simulink model "Bud3_wezel1_2010"  (R2024b)
settings: Solver=ode45  StartTime=0.0  StopTime=1000  MaxStep=0.1  RelTol=1e-3  EnableMultiTasking=on
values from neighbouring files (symbols this model uses):
  atz_c = (TwzN-TzewN)/(TwewN-TzewN)    (= 3.75)    [project1.m]
  btz_c = (TwzN-TwewN)/(TwewN-TzewN)    (= 2.75)    [project1.m]
  cpw = 4200    [project1.m]
  Cw = cpw*row*Vw  / skala    (= 700)    [project1.m]
  czas_skok = 100    [project1.m]
  dFg = [0, 0, 0] .* FgN    [project1.m]
  dFw = 0.1 * FwN    [project1.m]
  dQd = [0, 0, 0] .* QN    [project1.m]
  dSPc = 0    [project1.m]
  dTwz = 0    [project1.m]
  dTzew = 0    [project1.m]
  Fg0 = [1, 1, 1] .* FgN    [project1.m]
  Fw0 = tabFw0(ipp)    [project1.m]
  k = 1 / (0.1*FwN)    [project1.m]
  Kco = QwN / (TwpN - TozN)    [project1.m]
  KPc = 1    [project1.m]
  Qd0 = [0, 0, 0]    [project1.m]
  SPc0 = TwewN    (= 20)    [project1.m]
  T = 1000    [project1.m]
  T0 = 100    [project1.m]
  tau_cieplownia = 60*60 / skala    (= 60)    [project1.m]
  Tgp032 = (Tgp0(3)*Fg0(3) + Tgp0(2)*Fg0(2)  )   /   (  Fg0(3)+Fg0(2)    )    [project1.m]
  Tgp0321 = (Tgp0(3)*Fg0(3) + Tgp0(2)*Fg0(2)  + Tgp0(1)*Fg0(1)  )   /   (  Fg0(3) + Fg0(2) + Fg0(1)    )    [project1.m]
  Toz0 = x0( IlePom*2+1)    [project1.m]
  Twp0 = x0( IlePom*2+2)    [project1.m]
  Twz0 = tabTwz0(ipp)    [project1.m]
  Tzew0 = tabTzew0(ipp)    [project1.m]
undefined symbols (not defined in the file or in its folder): Cg, Cp, Kg, Kstr, T0_s, Tgp0, Twew0
settings Model: Creator=Mateusz  LastModifiedBy=Adam
settings SolverCC: AlgebraicLoopSolver=TrustRegion
settings DataIOCC: LimitDataPoints=on  SaveFormat=Array  SignalLoggingSaveFormat=ModelDataLogs  ReturnWorkspaceOutputs=off
settings OptimizationCC: ExpressionDepthLimit=2147483647  LifeSpan=inf
settings DebuggingCC: UnderspecifiedInitializationDetection=Classic  MergeDetectMultiDrivingBlocksExec=none  SolverPrmCheckMsg=warning  FcnCallInpInsideContextMsg=warning  UnconnectedInputMsg=warning  UnconnectedOutputMsg=warning  UnconnectedLineMsg=warning  StateNameClashWarn=warning  SFUnexpectedBacktrackingDiag=warning  SFNoUnconditionalDefaultTransitionDiag=warning  SFExecutionAtInitializationDiag=none  ArithmeticOperatorsInVariantConditions=warning
settings HardwareCC: ProdBitPerPointer=32  ProdBitPerSizeT=32  ProdBitPerPtrDiffT=32  ProdLargestAtomicFloat=None  ProdIntDivRoundTo=Undefined  ProdEndianess=Unspecified  ProdWordSize=32  ProdHWDeviceType=32-bit Generic
settings ModelReferenceCC: PropagateSignalLabelsOutOfModel=off
settings SFSimCC: SimUseLocalCustomCode=off  CustomCodeUndefinedFunction=UseInterfaceOnly
settings RTWCC: RTWUseLocalCustomCode=off  GPUComputeCapability=3.5
settings CodeAppCC: StateflowObjectComments=on
settings GRTTargetCC: TargetLangStandard=C89/C90 (ANSI)  CombineOutputUpdateFcns=off  GRTInterface=on
settings ConfigComp: CovMetricSettings=dw  CovSaveCumulativeToWorkspaceVar=on  CovSaveSingleToWorkspaceVar=on  CovExternalEMLEnable=off

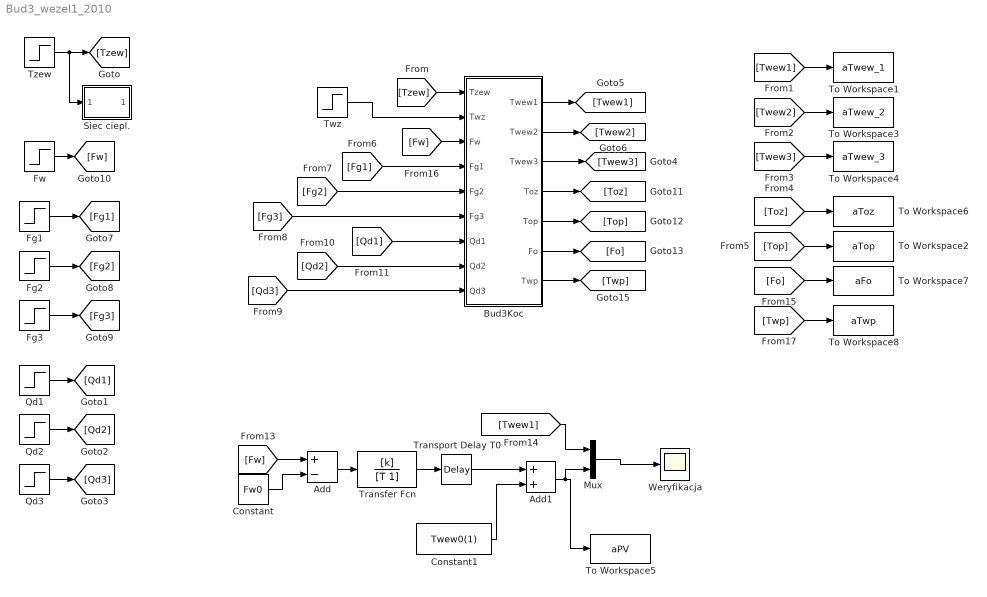
== system Bud3_wezel1_2010 ==
  Add : Sum  Inputs=+-
  Add1 : Sum
  Bud3Koc : Subsystem
  Constant : Constant  Value=Fw0
  Constant1 : Constant  Value=Twew0(1)
  Fg1 : Step  Time=czas_skok  Before=Fg0(1)  After=Fg0(1)+dFg(1)  SampleTime=0
  Fg2 : Step  Time=czas_skok  Before=Fg0(2)  After=Fg0(2)+dFg(2)  SampleTime=0
  Fg3 : Step  Time=czas_skok  Before=Fg0(3)  After=Fg0(3)+dFg(3)  SampleTime=0
  Fw : Step  Time=czas_skok  Before=Fw0  After=Fw0+dFw  SampleTime=0
  Mux : Mux  Inputs=2
  Qd1 : Step  Time=czas_skok  Before=Qd0(1)  After=Qd0(1)+dQd(1)  SampleTime=0
  Qd2 : Step  Time=czas_skok  Before=Qd0(2)  After=Qd0(2)+dQd(2)  SampleTime=0
  Qd3 : Step  Time=czas_skok  Before=Qd0(3)  After=Qd0(3)+dQd(3)  SampleTime=0
  Siec ciepl. : Subsystem
  To Workspace1 : ToWorkspace  VariableName=aTwew_1  SampleTime=-1
  To Workspace2 : ToWorkspace  VariableName=aTop  SampleTime=-1
  To Workspace3 : ToWorkspace  VariableName=aTwew_2  SampleTime=-1
  To Workspace4 : ToWorkspace  VariableName=aTwew_3  SampleTime=-1
  To Workspace5 : ToWorkspace  VariableName=aPV  SampleTime=-1
  To Workspace6 : ToWorkspace  VariableName=aToz  SampleTime=-1
  To Workspace7 : ToWorkspace  VariableName=aFo  SampleTime=-1
  To Workspace8 : ToWorkspace  VariableName=aTwp  SampleTime=-1
  Transfer Fcn : TransferFcn  Numerator=[k]  Denominator=[T 1]
  Transport Delay T0 : TransportDelay  DelayTime=T0
  Twz : Step  Time=czas_skok  Before=Twz0  After=Twz0 + dTwz  SampleTime=0
  Tzew : Step  Time=czas_skok  Before=Tzew0  After=Tzew0+dTzew  SampleTime=0
  Weryfikacja : Scope
  wires:
  Tzew/1 -> [Tzew], Siec ciepl./1(Tzew)
  Fg1/1 -> [Fg1]
  Fg2/1 -> [Fg2]
  Fg3/1 -> [Fg3]
  Fw/1 -> [Fw]
  Transfer Fcn/1 -> Transport Delay T0/1
  Add/1 -> Transfer Fcn/1
  [Fw] -> Add/1
  Constant/1 -> Add/2
  [Twew1] -> Mux/1
  Mux/1 -> Weryfikacja/1
  Transport Delay T0/1 -> Add1/1
  Add1/1 -> Mux/2, To Workspace5/1
  Constant1/1 -> Add1/2
  Bud3Koc/1(Twew1) -> [Twew1]
  Bud3Koc/2(Twew2) -> [Twew2]
  Twz/1 -> Bud3Koc/2(Twz)
  [Tzew] -> Bud3Koc/1(Tzew)
  [Fg1] -> Bud3Koc/4(Fg1)
  [Fg2] -> Bud3Koc/5(Fg2)
  [Fg3] -> Bud3Koc/6(Fg3)
  Qd1/1 -> [Qd1]
  Qd2/1 -> [Qd2]
  Qd3/1 -> [Qd3]
  [Twew1] -> To Workspace1/1
  [Twew2] -> To Workspace3/1
  [Twew3] -> To Workspace4/1
  Bud3Koc/4(Toz) -> [Toz]
  Bud3Koc/5(Top) -> [Top]
  [Toz] -> To Workspace6/1
  [Top] -> To Workspace2/1
  [Qd3] -> Bud3Koc/9(Qd3)
  [Qd2] -> Bud3Koc/8(Qd2)
  [Qd1] -> Bud3Koc/7(Qd1)
  Bud3Koc/6(Fo) -> [Fo]
  [Fo] -> To Workspace7/1
  Bud3Koc/3(Twew3) -> [Twew3]
  [Fw] -> Bud3Koc/3(Fw)
  [Twp] -> To Workspace8/1
  Bud3Koc/7(Twp) -> [Twp]

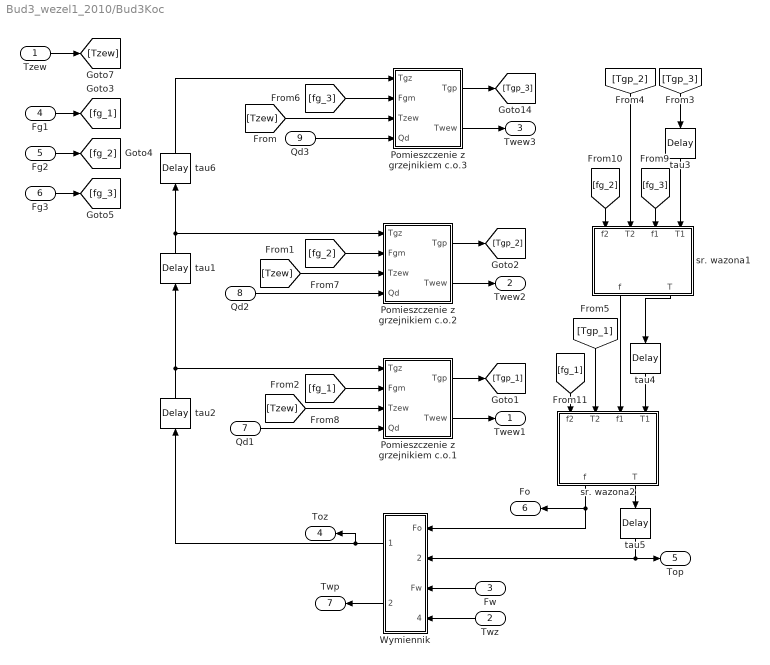
== system Bud3_wezel1_2010/Bud3Koc ==
  Tzew : Inport
  Twz : Inport  Port=2
  Fw : Inport  Port=3
  Fg1 : Inport  Port=4
  Fg2 : Inport  Port=5
  Fg3 : Inport  Port=6
  Qd1 : Inport  Port=7
  Qd2 : Inport  Port=8
  Qd3 : Inport  Port=9
  Pomieszczenie z grzejnikiem c.o.1 : Subsystem  mask{kg=Kg(1), kstr=Kstr(1), Cg=Cg(1), Cp=Cp(1), Tgp0=Tgp0(1), Twew0=Twew0(1), cpw=cpw}
      mask prompts: kg "Wspolczynnik strat ciepla scian grzejnika"; kstr "Wspolczynnik strat ciepla scian pomieszczenia"; Cg "Pojemnosc cieplna grzejnika"; Cp "Pojemnosc cieplna pomieszczenia"; Tgp0 "Temperatura poczatkowa wody powracajacej"; Twew0 "Temperatura poczatkowa wewnatrz pomieszczenia"; cpw "Cieplo wlasciwe"
      mask init:
      | cpw=4200;
      | row=1000;
  Pomieszczenie z grzejnikiem c.o.2 : Subsystem  mask{kg=Kg(2), kstr=Kstr(2), Cg=Cg(2), Cp=Cp(2), Tgp0=Tgp0(2), Twew0=Twew0(2), cpw=cpw}
      mask prompts: kg "Wspolczynnik strat ciepla scian grzejnika"; kstr "Wspolczynnik strat ciepla scian pomieszczenia"; Cg "Pojemnosc cieplna grzejnika"; Cp "Pojemnosc cieplna pomieszczenia"; Tgp0 "Temperatura poczatkowa wody powracajacej"; Twew0 "Temperatura poczatkowa wewnatrz pomieszczenia"; cpw "Cieplo wlasciwe"
      mask init:
      | cpw=4200;
      | row=1000;
  Pomieszczenie z grzejnikiem c.o.3 : Subsystem  mask{kg=Kg(3), kstr=Kstr(3), Cg=Cg(3), Cp=Cp(3), Tgp0=Tgp0(3), Twew0=Twew0(3), cpw=cpw}
      mask prompts: kg "Wspolczynnik strat ciepla scian grzejnika"; kstr "Wspolczynnik strat ciepla scian pomieszczenia"; Cg "Pojemnosc cieplna grzejnika"; Cp "Pojemnosc cieplna pomieszczenia"; Tgp0 "Temperatura poczatkowa wody powracajacej"; Twew0 "Temperatura poczatkowa wewnatrz pomieszczenia"; cpw "Cieplo wlasciwe"
      mask init:
      | cpw=4200;
      | row=1000;
  Wymiennik : Subsystem  mask{cpw=cpw, Kcc=Kco, Cv1=Cw, Cv2=Cw, Twp0=Twp0, Toz0=Toz0}
      mask prompts: Cv1 "Cv1 (str.zasilania)"; Cv2 "Cv2 (str.odbiornik)"
  sr. wazona1 : Subsystem
  sr. wazona2 : Subsystem
  tau1 : TransportDelay  DelayTime=T0_s(2)  InitialOutput=Toz0
  tau2 : TransportDelay  DelayTime=T0_s(1)  InitialOutput=Toz0
  tau3 : TransportDelay  DelayTime=T0_s(3)  InitialOutput=Tgp0(3)
  tau4 : TransportDelay  DelayTime=T0_s(2)  InitialOutput=Tgp032
  tau5 : TransportDelay  DelayTime=T0_s(1)  InitialOutput=Tgp0321
  tau6 : TransportDelay  DelayTime=T0_s(3)  InitialOutput=Toz0
  Twew1 : Outport
  Twew2 : Outport  Port=2
  Twew3 : Outport  Port=3
  Toz : Outport  Port=4
  Top : Outport  Port=5
  Fo : Outport  Port=6
  Twp : Outport  Port=7
  wires:
  tau1/1 -> Pomieszczenie z grzejnikiem c.o.2/1(Tgz), tau6/1
  tau2/1 -> Pomieszczenie z grzejnikiem c.o.1/1(Tgz), tau1/1
  Wymiennik/1(Toz) -> tau2/1, Toz/1
  Qd2/1 -> Pomieszczenie z grzejnikiem c.o.2/4(Qd)
  sr. wazona1/2(T) -> tau4/1
  tau3/1 -> sr. wazona1/4(T1)
  sr. wazona2/2(T) -> tau5/1
  tau5/1 -> Top/1, Wymiennik/2(Top)
  sr. wazona2/1(f) -> Fo/1, Wymiennik/1(Fo)
  tau4/1 -> sr. wazona2/4(T1)
  sr. wazona1/1(f) -> sr. wazona2/3(f1)
  [Tzew] -> Pomieszczenie z grzejnikiem c.o.2/3(Tzew)
  Pomieszczenie z grzejnikiem c.o.1/1(Tgp) -> [Tgp_1]
  Pomieszczenie z grzejnikiem c.o.2/1(Tgp) -> [Tgp_2]
  [Tgp_3] -> tau3/1
  [Tgp_2] -> sr. wazona1/2(T2)
  [Tgp_1] -> sr. wazona2/2(T2)
  [fg_3] -> sr. wazona1/3(f1)
  [fg_2] -> sr. wazona1/1(f2)
  [fg_1] -> sr. wazona2/1(f2)
  Tzew/1 -> [Tzew]
  Pomieszczenie z grzejnikiem c.o.1/2(Twew) -> Twew1/1
  Pomieszczenie z grzejnikiem c.o.2/2(Twew) -> Twew2/1
  Qd1/1 -> Pomieszczenie z grzejnikiem c.o.1/4(Qd)
  [Tzew] -> Pomieszczenie z grzejnikiem c.o.1/3(Tzew)
  Pomieszczenie z grzejnikiem c.o.3/1(Tgp) -> [Tgp_3]
  Pomieszczenie z grzejnikiem c.o.3/2(Twew) -> Twew3/1
  Qd3/1 -> Pomieszczenie z grzejnikiem c.o.3/4(Qd)
  [Tzew] -> Pomieszczenie z grzejnikiem c.o.3/3(Tzew)
  tau6/1 -> Pomieszczenie z grzejnikiem c.o.3/1(Tgz)
  Fg1/1 -> [fg_1]
  Fg2/1 -> [fg_2]
  Fg3/1 -> [fg_3]
  [fg_3] -> Pomieszczenie z grzejnikiem c.o.3/2(Fgm)
  [fg_2] -> Pomieszczenie z grzejnikiem c.o.2/2(Fgm)
  [fg_1] -> Pomieszczenie z grzejnikiem c.o.1/2(Fgm)
  Wymiennik/2(Twp) -> Twp/1
  Fw/1 -> Wymiennik/3(Fw)
  Twz/1 -> Wymiennik/4(Twz)

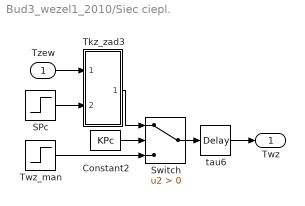
== system Bud3_wezel1_2010/Siec ciepl. ==
  Tzew : Inport
  Constant2 : Constant  Value=KPc
  SPc : Step  Time=czas_skok  Before=SPc0  After=SPc0+dSPc  SampleTime=0
  Switch : Switch  Criteria=u2 > Threshold  SaturateOnIntegerOverflow=off  InputSameDT=off
  Tkz_zad3 : Subsystem  mask{atp=atz_c, btp=btz_c}
      mask prompts: atp "atp (*Tw)"; btp "btp (*Tz)"
  Twz_man : Step  Time=czas_skok  Before=Twz0  After=Twz0+dTwz  SampleTime=0
  tau6 : TransportDelay  DelayTime=tau_cieplownia  InitialOutput=Twz0
  Twz : Outport
  wires:
  SPc/1 -> Tkz_zad3/2(Tw_zad)
  Tkz_zad3/1(Tsz) -> Switch/1
  Twz_man/1 -> Switch/3
  Constant2/1 -> Switch/2
  Switch/1 -> tau6/1
  Tzew/1 -> Tkz_zad3/1(Tzew)
  tau6/1 -> Twz/1

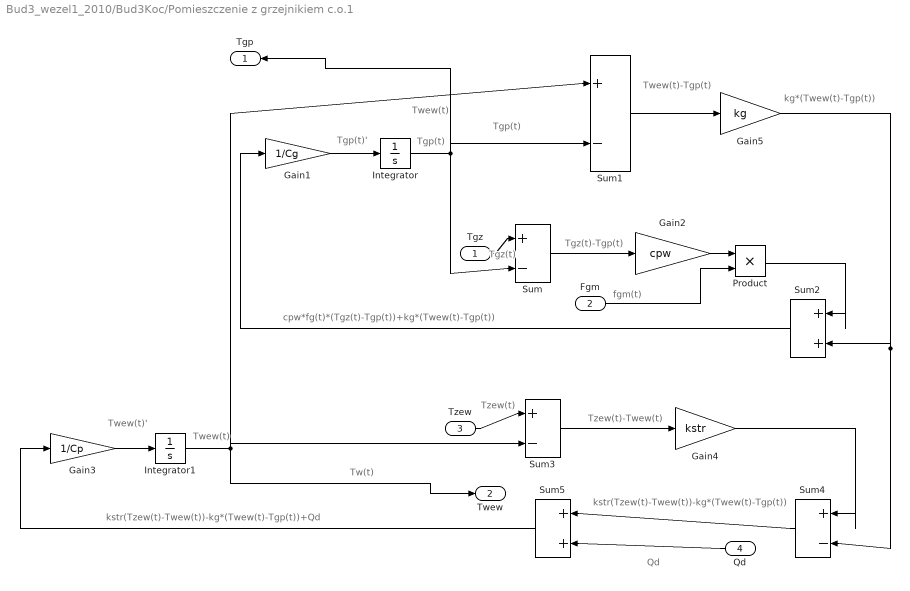
== system Bud3_wezel1_2010/Bud3Koc/Pomieszczenie z grzejnikiem c.o.1 ==
  note: Tgp(t)'
  note: Tgp(t)
  note: Tgz(t)-Tgp(t)
  note: fgm(t)
  note: Tgz(t)
  note: Twew(t)'
  note: Twew(t)
  note: Tzew(t)-Twew(t)
  note: Tzew(t)
  note: Twew(t)-Tgp(t)
  note: Twew(t)
  note: Tw(t)
  note: Tgp(t)
  note: Qd
  note: kg*(Twew(t)-Tgp(t))
  note: cpw*fg(t)*(Tgz(t)-Tgp(t))+kg*(Twew(t)-Tgp(t))
  note: kstr(Tzew(t)-Twew(t))-kg*(Twew(t)-Tgp(t))
  note: kstr(Tzew(t)-Twew(t))-kg*(Twew(t)-Tgp(t))+Qd
  Tgz : Inport
  Fgm : Inport  Port=2
  Tzew : Inport  Port=3
  Qd : Inport  Port=4
  Gain1 : Gain  Gain=1/Cg
  Gain2 : Gain  Gain=cpw
  Gain3 : Gain  Gain=1/Cp
  Gain4 : Gain  Gain=kstr
  Gain5 : Gain  Gain=kg
  Integrator : Integrator  InitialCondition=Tgp0
  Integrator1 : Integrator  InitialCondition=Twew0
  Product : Product  RndMeth=Zero
  Sum{,1,3..4} (4 alike) : Sum  Inputs=|+-
  Sum2 : Sum  Inputs=|++
  Sum5 : Sum  Inputs=|++
  Tgp : Outport
  Twew : Outport  Port=2
  wires:
  Integrator/1 -> Sum/2, Sum1/2, Tgp/1
  Tgz/1 -> Sum/1
  Gain1/1 -> Integrator/1
  Sum/1 -> Gain2/1
  Sum1/1 -> Gain5/1
  Fgm/1 -> Product/2
  Integrator1/1 -> Sum1/1, Sum3/2, Twew/1
  Gain3/1 -> Integrator1/1
  Sum3/1 -> Gain4/1
  Gain5/1 -> Sum2/2, Sum4/2
  Tzew/1 -> Sum3/1
  Sum5/1 -> Gain3/1
  Sum2/1 -> Gain1/1
  Product/1 -> Sum2/1
  Gain4/1 -> Sum4/1
  Qd/1 -> Sum5/2
  Sum4/1 -> Sum5/1
  Gain2/1 -> Product/1

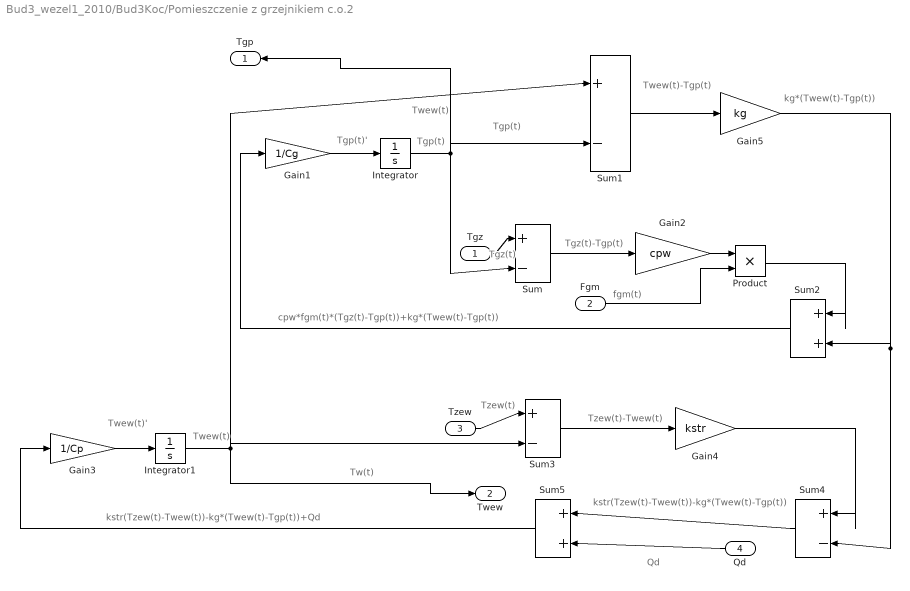
== system Bud3_wezel1_2010/Bud3Koc/Pomieszczenie z grzejnikiem c.o.2 ==
  note: Tgp(t)'
  note: Tgp(t)
  note: Tgz(t)-Tgp(t)
  note: fgm(t)
  note: Tgz(t)
  note: Twew(t)'
  note: Twew(t)
  note: Tzew(t)-Twew(t)
  note: Tzew(t)
  note: Twew(t)-Tgp(t)
  note: Twew(t)
  note: Tw(t)
  note: Tgp(t)
  note: Qd
  note: kg*(Twew(t)-Tgp(t))
  note: cpw*fgm(t)*(Tgz(t)-Tgp(t))+kg*(Twew(t)-Tgp(t))
  note: kstr(Tzew(t)-Twew(t))-kg*(Twew(t)-Tgp(t))
  note: kstr(Tzew(t)-Twew(t))-kg*(Twew(t)-Tgp(t))+Qd
  Tgz : Inport
  Fgm : Inport  Port=2
  Tzew : Inport  Port=3
  Qd : Inport  Port=4
  Gain1 : Gain  Gain=1/Cg
  Gain2 : Gain  Gain=cpw
  Gain3 : Gain  Gain=1/Cp
  Gain4 : Gain  Gain=kstr
  Gain5 : Gain  Gain=kg
  Integrator : Integrator  InitialCondition=Tgp0
  Integrator1 : Integrator  InitialCondition=Twew0
  Product : Product  RndMeth=Zero
  Sum{,1,3..4} (4 alike) : Sum  Inputs=|+-
  Sum2 : Sum  Inputs=|++
  Sum5 : Sum  Inputs=|++
  Tgp : Outport
  Twew : Outport  Port=2
  wires:
  Integrator/1 -> Sum/2, Sum1/2, Tgp/1
  Tgz/1 -> Sum/1
  Gain1/1 -> Integrator/1
  Sum/1 -> Gain2/1
  Sum1/1 -> Gain5/1
  Fgm/1 -> Product/2
  Integrator1/1 -> Sum1/1, Sum3/2, Twew/1
  Gain3/1 -> Integrator1/1
  Sum3/1 -> Gain4/1
  Gain5/1 -> Sum2/2, Sum4/2
  Tzew/1 -> Sum3/1
  Sum5/1 -> Gain3/1
  Sum2/1 -> Gain1/1
  Product/1 -> Sum2/1
  Gain4/1 -> Sum4/1
  Qd/1 -> Sum5/2
  Sum4/1 -> Sum5/1
  Gain2/1 -> Product/1

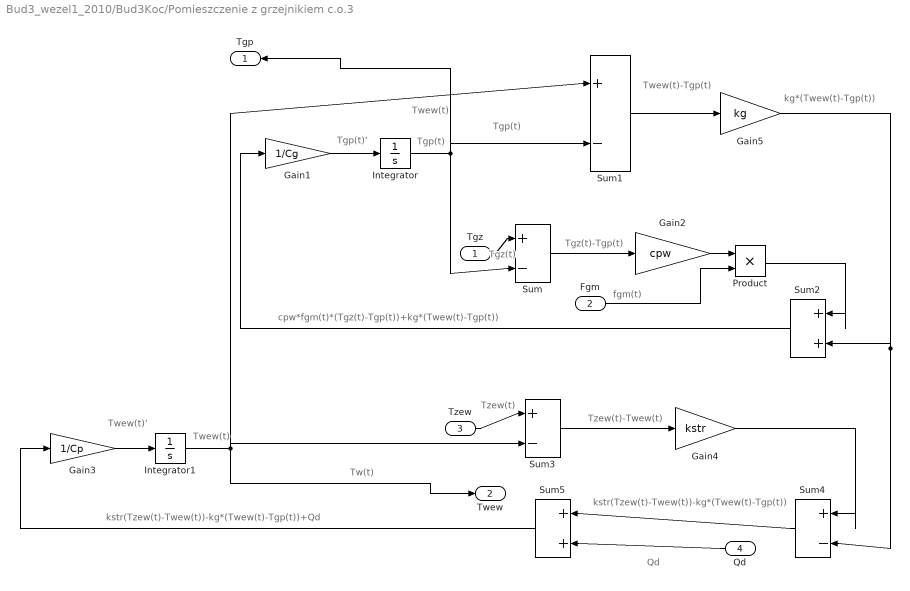
== system Bud3_wezel1_2010/Bud3Koc/Pomieszczenie z grzejnikiem c.o.3 ==
  note: Tgp(t)'
  note: Tgp(t)
  note: Tgz(t)-Tgp(t)
  note: fgm(t)
  note: Tgz(t)
  note: Twew(t)'
  note: Twew(t)
  note: Tzew(t)-Twew(t)
  note: Tzew(t)
  note: Twew(t)-Tgp(t)
  note: Twew(t)
  note: Tw(t)
  note: Tgp(t)
  note: Qd
  note: kg*(Twew(t)-Tgp(t))
  note: cpw*fgm(t)*(Tgz(t)-Tgp(t))+kg*(Twew(t)-Tgp(t))
  note: kstr(Tzew(t)-Twew(t))-kg*(Twew(t)-Tgp(t))
  note: kstr(Tzew(t)-Twew(t))-kg*(Twew(t)-Tgp(t))+Qd
  Tgz : Inport
  Fgm : Inport  Port=2
  Tzew : Inport  Port=3
  Qd : Inport  Port=4
  Gain1 : Gain  Gain=1/Cg
  Gain2 : Gain  Gain=cpw
  Gain3 : Gain  Gain=1/Cp
  Gain4 : Gain  Gain=kstr
  Gain5 : Gain  Gain=kg
  Integrator : Integrator  InitialCondition=Tgp0
  Integrator1 : Integrator  InitialCondition=Twew0
  Product : Product  RndMeth=Zero
  Sum{,1,3..4} (4 alike) : Sum  Inputs=|+-
  Sum2 : Sum  Inputs=|++
  Sum5 : Sum  Inputs=|++
  Tgp : Outport
  Twew : Outport  Port=2
  wires:
  Integrator/1 -> Sum/2, Sum1/2, Tgp/1
  Tgz/1 -> Sum/1
  Gain1/1 -> Integrator/1
  Sum/1 -> Gain2/1
  Sum1/1 -> Gain5/1
  Fgm/1 -> Product/2
  Integrator1/1 -> Sum1/1, Sum3/2, Twew/1
  Gain3/1 -> Integrator1/1
  Sum3/1 -> Gain4/1
  Gain5/1 -> Sum2/2, Sum4/2
  Tzew/1 -> Sum3/1
  Sum5/1 -> Gain3/1
  Sum2/1 -> Gain1/1
  Product/1 -> Sum2/1
  Gain4/1 -> Sum4/1
  Qd/1 -> Sum5/2
  Sum4/1 -> Sum5/1
  Gain2/1 -> Product/1

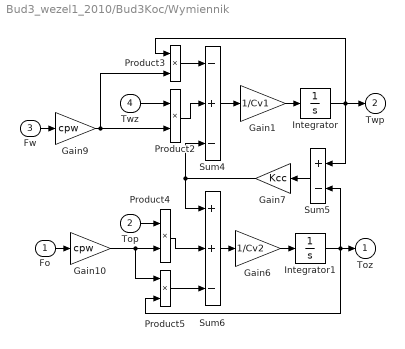
== system Bud3_wezel1_2010/Bud3Koc/Wymiennik ==
  Fo : Inport
  Top : Inport  Port=2
  Fw : Inport  Port=3
  Twz : Inport  Port=4
  Gain1 : Gain  Gain=1/Cv1  SaturateOnIntegerOverflow=on  OutDataTypeStr=Inherit: Same as input  ParamDataTypeStr=Inherit: Same as input
  Gain10 : Gain  Gain=cpw  SaturateOnIntegerOverflow=on  OutDataTypeStr=Inherit: Same as input  ParamDataTypeStr=Inherit: Same as input
  Gain6 : Gain  Gain=1/Cv2  SaturateOnIntegerOverflow=on  OutDataTypeStr=Inherit: Same as input  ParamDataTypeStr=Inherit: Same as input
  Gain7 : Gain  Gain=Kcc  SaturateOnIntegerOverflow=on  OutDataTypeStr=Inherit: Same as input  ParamDataTypeStr=Inherit: Same as input
  Gain9 : Gain  Gain=cpw  SaturateOnIntegerOverflow=on  OutDataTypeStr=Inherit: Same as input  ParamDataTypeStr=Inherit: Same as input
  Integrator : Integrator  InitialCondition=Twp0
  Integrator1 : Integrator  InitialCondition=Toz0
  Product{2..5} (4 alike) : Product  Inputs=**  InputSameDT=on  RndMeth=Zero  SaturateOnIntegerOverflow=on  OutDataTypeStr=Inherit: Same as first input
  Sum4 : Sum  Inputs=-+-  InputSameDT=on  SaturateOnIntegerOverflow=on  OutDataTypeStr=Inherit: Same as first input
  Sum5 : Sum  Inputs=+-  InputSameDT=on  SaturateOnIntegerOverflow=on  OutDataTypeStr=Inherit: Same as first input
  Sum6 : Sum  Inputs=++-  InputSameDT=on  SaturateOnIntegerOverflow=on  OutDataTypeStr=Inherit: Same as first input
  Toz : Outport
  Twp : Outport  Port=2
  wires:
  Product3/1 -> Sum4/1
  Product2/1 -> Sum4/2
  Twz/1 -> Product2/1
  Fw/1 -> Gain9/1
  Gain9/1 -> Product2/2, Product3/2
  Sum4/1 -> Gain1/1
  Gain1/1 -> Integrator/1
  Integrator/1 -> Twp/1, Product3/1, Sum5/1
  Sum6/1 -> Gain6/1
  Gain6/1 -> Integrator1/1
  Sum5/1 -> Gain7/1
  Integrator1/1 -> Toz/1, Sum5/2, Product5/2
  Gain7/1 -> Sum4/3, Sum6/1
  Product4/1 -> Sum6/2
  Product5/1 -> Sum6/3
  Fo/1 -> Gain10/1
  Top/1 -> Product4/1
  Gain10/1 -> Product4/2, Product5/1

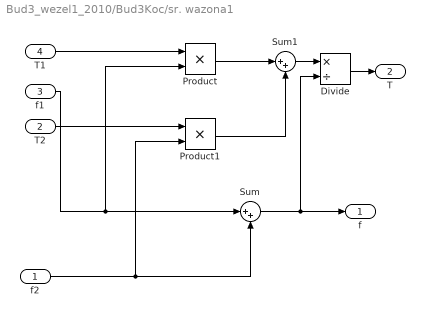
== system Bud3_wezel1_2010/Bud3Koc/sr. wazona1 ==
  f2 : Inport
  T2 : Inport  Port=2
  f1 : Inport  Port=3
  T1 : Inport  Port=4
  Divide : Product  Inputs=*/
  Product : Product  RndMeth=Zero
  Product1 : Product  RndMeth=Zero
  Sum : Sum  Inputs=|++
  Sum1 : Sum  Inputs=|++
  f : Outport
  T : Outport  Port=2
  wires:
  T1/1 -> Product/1
  T2/1 -> Product1/1
  f1/1 -> Product/2, Sum/1
  f2/1 -> Product1/2, Sum/2
  Product/1 -> Sum1/1
  Product1/1 -> Sum1/2
  Sum/1 -> f/1, Divide/2
  Sum1/1 -> Divide/1
  Divide/1 -> T/1

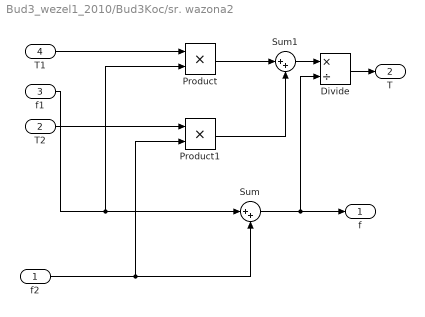
== system Bud3_wezel1_2010/Bud3Koc/sr. wazona2 ==
  f2 : Inport
  T2 : Inport  Port=2
  f1 : Inport  Port=3
  T1 : Inport  Port=4
  Divide : Product  Inputs=*/
  Product : Product  RndMeth=Zero
  Product1 : Product  RndMeth=Zero
  Sum : Sum  Inputs=|++
  Sum1 : Sum  Inputs=|++
  f : Outport
  T : Outport  Port=2
  wires:
  T1/1 -> Product/1
  T2/1 -> Product1/1
  f1/1 -> Product/2, Sum/1
  f2/1 -> Product1/2, Sum/2
  Product/1 -> Sum1/1
  Product1/1 -> Sum1/2
  Sum/1 -> f/1, Divide/2
  Sum1/1 -> Divide/1
  Divide/1 -> T/1

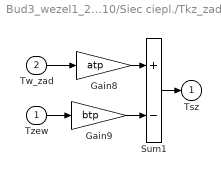
== system Bud3_wezel1_2010/Siec ciepl./Tkz_zad3 ==
  Tzew : Inport
  Tw_zad : Inport  Port=2
  Gain8 : Gain  Gain=atp  SaturateOnIntegerOverflow=on  OutDataTypeStr=Inherit: Same as input  ParamDataTypeStr=Inherit: Same as input
  Gain9 : Gain  Gain=btp  SaturateOnIntegerOverflow=on  OutDataTypeStr=Inherit: Same as input  ParamDataTypeStr=Inherit: Same as input
  Sum1 : Sum  Inputs=+-  InputSameDT=on  SaturateOnIntegerOverflow=on  OutDataTypeStr=Inherit: Same as first input
  Tsz : Outport
  wires:
  Tw_zad/1 -> Gain8/1
  Gain8/1 -> Sum1/1
  Gain9/1 -> Sum1/2
  Tzew/1 -> Gain9/1
  Sum1/1 -> Tsz/1
